simulink model "QuadCarModel"  (R2019b)
settings: Solver=VariableStepAuto  StartTime=0.0  StopTime=10.0  RelTol=1e-3
undefined symbols (not defined in the file or in its folder): Cs, Ks, Kt, M, Mu
settings Model: Creator=ip  LastModifiedBy=ip

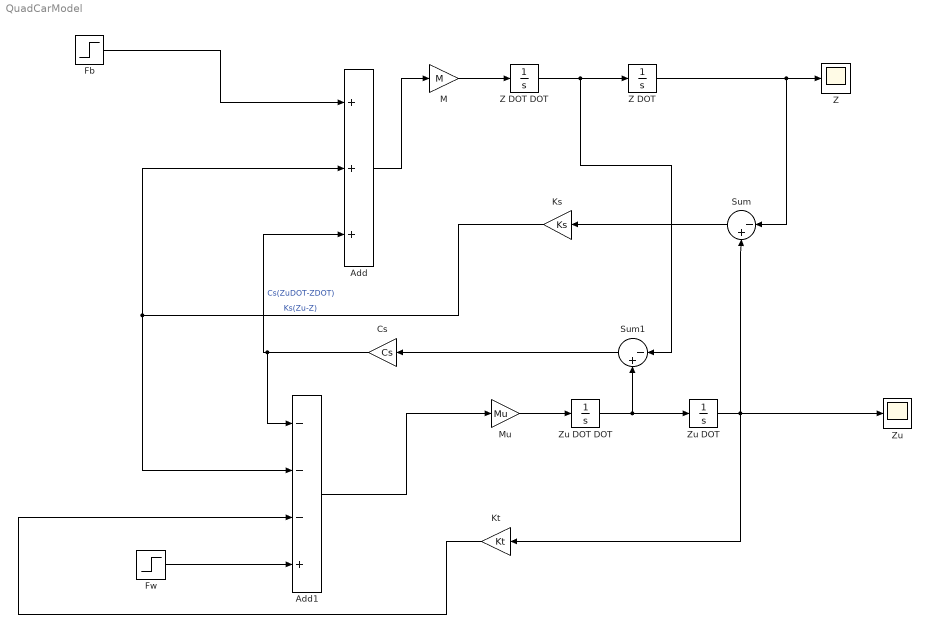
== system QuadCarModel ==
  Add : Sum  Inputs=+++
  Add1 : Sum  Inputs=---+
  Cs : Gain  Gain=Cs
  Fb : Step  SampleTime=0
  Fw : Step  SampleTime=0
  Ks : Gain  Gain=Ks
  Kt : Gain  Gain=Kt
  M : Gain  Gain=M
  Mu : Gain  Gain=Mu
  Sum : Sum  Inputs=|-+
  Sum1 : Sum  Inputs=|-+
  Z : Scope
  Z DOT : Integrator
  Z DOT DOT : Integrator
  Zu : Scope
  Zu DOT : Integrator
  Zu DOT DOT : Integrator
  wires:
  Z DOT DOT/1 -> Sum1/1, Z DOT/1
  Z DOT/1 -> Sum/1, Z/1
  M/1 -> Z DOT DOT/1
  Add/1 -> M/1
  Fb/1 -> Add/1
  Mu/1 -> Zu DOT DOT/1
  Zu DOT/1 -> Kt/1, Zu/1, Sum/2
  Zu DOT DOT/1 -> Zu DOT/1, Sum1/2
  Sum/1 -> Ks/1
  Ks/1 -> Add1/2, Add/2  "Ks(Zu-Z)"
  Cs/1 -> Add1/1, Add/3  "Cs(ZuDOT-ZDOT)"
  Sum1/1 -> Cs/1
  Kt/1 -> Add1/3
  Add1/1 -> Mu/1
  Fw/1 -> Add1/4
